simulink model "Copy_2_of_SUS_ST_GUI"  (R2013a)
settings: Solver=ode3  StartTime=0  StopTime=T  FixedStep=0.1  RelTol=1e-3
values from neighbouring files (symbols this model uses):
  CA = str2double(get(handles.CA,'string'))    [SUS_ST_0326.m]    (also in SUS_ST_GUI_0326.m)
  IN = str2double(get(handles.IN,'string'))    [SUS_ST_0326.m]    (also in SUS_ST_GUI_0326.m)
  LT = str2double(get(handles.LT,'string'))    [SUS_ST_GUI_0326.m]
  N = 1    [SUS_ST_0326.m]
  SR = str2double(get(handles.SR,'string'))    [SUS_ST_0326.m]    (also in SUS_ST_GUI_0326.m)
  ST = str2double(get(handles.ST,'string'))    [SUS_ST_GUI_0326.m]
  ST_S = str2double(get(handles.ST_S,'string'))    [SUS_ST_GUI_0326.m]
  T = 10    [SUS_ST_GUI_0326.m]
  T5 = str2double(get(handles.T5,'string'))    [SUS_ST_0326.m]    (also in SUS_ST_GUI_0326.m)
  T6 = str2double(get(handles.T6,'string'))    [SUS_ST_0326.m]    (also in SUS_ST_GUI_0326.m)
  X11 = (Z11-H/sind(CA)-b2_3)/k2_3    [SUS_ST_GUI_0326.m]
  X12 = (Z12-bb2_3)/k2_3    [SUS_ST_GUI_0326.m]
  X13 = X12-X12_3    [SUS_ST_GUI_0326.m]
  X14 = X9+X14_1    [SUS_ST_GUI_0326.m]
  X15 = X9+X15_1    [SUS_ST_GUI_0326.m]
  X16 = X9+X16_2    [SUS_ST_GUI_0326.m]
  X2 = -abs(Z3)*tand(CA)    [SUS_ST_GUI_0326.m]
  x2 = 0    [SUS_ST_GUI_0326.m]
  X3 = abs(Z2)*tand(CA)    [SUS_ST_GUI_0326.m]
  x3 = 0    [SUS_ST_GUI_0326.m]
  x4 = str2double(get(handles.x4,'string'))    [SUS_ST_0326.m]    (also in SUS_ST_GUI_0326.m)
  X5 = X4-a1*cosd(T5)    [SUS_ST_GUI_0326.m]
  x5 = 0    [SUS_ST_GUI_0326.m]
  X6 = X4+b1*cosd(T5)    [SUS_ST_GUI_0326.m]
  x6 = str2double(get(handles.x6,'string'))    [SUS_ST_0326.m]    (also in SUS_ST_GUI_0326.m)
  X7 = X1-a2*cosd(T6)    [SUS_ST_GUI_0326.m]
  x7 = x4-e7    [SUS_ST_GUI_0326.m]
  X8 = X1+b2*cosd(T6)    [SUS_ST_GUI_0326.m]
  x8 = x9-l8*sind(t8)    [SUS_ST_GUI_0326.m]
  X9 = str2double(get(handles.X9,'string'))    [SUS_ST_0326.m]    (also in SUS_ST_GUI_0326.m)
  x9 = str2double(get(handles.x9,'string'))    [SUS_ST_0326.m]    (also in SUS_ST_GUI_0326.m)
  XC1 = (X7+X2+X8)/3    [SUS_ST_GUI_0326.m]
  xc1 = (x3+x4+x5)/3    [SUS_ST_GUI_0326.m]
  XC2 = (X3+X2)/2    [SUS_ST_GUI_0326.m]
  XC3 = (X5+X3+X6)/3    [SUS_ST_GUI_0326.m]
  Y11 = M/2    [SUS_ST_GUI_0326.m]
  Y12 = (B11_12-BB2_3)/(K2_3-K11_12)    [SUS_ST_GUI_0326.m]
  Y13 = Y12-Y12_3    [SUS_ST_GUI_0326.m]
  Y14 = Y9+Y14_1    [SUS_ST_GUI_0326.m]
  Y15 = Y9+Y15_1    [SUS_ST_GUI_0326.m]
  Y16 = Y9+Y16_2    [SUS_ST_GUI_0326.m]
  Y2 = (Z2-Z9)/K2_3+Y9-SR    [SUS_ST_GUI_0326.m]
  y2 = Y1+l2*cosd(t2+T2)    [SUS_ST_GUI_0326.m]
  Y3 = (Z3-Z9)/K2_3+Y9-SR    [SUS_ST_GUI_0326.m]
  y3 = y4+l4*cosd(t4)    [SUS_ST_GUI_0326.m]
  y4 = str2double(get(handles.y4,'string'))    [SUS_ST_0326.m]    (also in SUS_ST_GUI_0326.m)
  Y5 = Y4    [SUS_ST_GUI_0326.m]
  y5 = y4+l5*cosd(t5)    [SUS_ST_GUI_0326.m]
  Y6 = Y4    [SUS_ST_GUI_0326.m]
  y6 = str2double(get(handles.y6,'string'))    [SUS_ST_0326.m]    (also in SUS_ST_GUI_0326.m)
  Y7 = Y1    [SUS_ST_GUI_0326.m]
  y7 = y4+l7*cosd(t7)    [SUS_ST_GUI_0326.m]
  Y8 = Y1    [SUS_ST_GUI_0326.m]
  y8 = y9+l8*cosd(t8)    [SUS_ST_GUI_0326.m]
  Y9 = str2double(get(handles.Y9,'string'))    [SUS_ST_0326.m]    (also in SUS_ST_GUI_0326.m)
  y9 = str2double(get(handles.y9,'string'))    [SUS_ST_0326.m]    (also in SUS_ST_GUI_0326.m)
  YC1 = (Y7+Y2+Y8)/3    [SUS_ST_GUI_0326.m]
  yc1 = (y3+y4+y5)/3    [SUS_ST_GUI_0326.m]
  YC2 = (Y3+Y2)/2    [SUS_ST_GUI_0326.m]
  YC3 = (Y5+Y3+Y6)/3    [SUS_ST_GUI_0326.m]
  Z11 = str2double(get(handles.Z11,'string'))    [SUS_ST_0326.m]    (also in SUS_ST_GUI_0326.m)
  Z12 = str2double(get(handles.Z12,'string'))    [SUS_ST_0326.m]    (also in SUS_ST_GUI_0326.m = K11_12*Y12+B11_12)
  Z13 = Z12-Z12_3    [SUS_ST_GUI_0326.m]
  Z14 = Z9+Z14_1    [SUS_ST_GUI_0326.m]
  Z15 = Z9+Z15_1    [SUS_ST_GUI_0326.m]
  Z16 = Z9+Z16_2    [SUS_ST_GUI_0326.m]
  Z2 = str2double(get(handles.Z2,'string'))    [SUS_ST_0326.m]    (also in SUS_ST_GUI_0326.m)
  z2 = Z1+l2*sind(t2+T2)    [SUS_ST_GUI_0326.m]
  Z3 = str2double(get(handles.Z3,'string'))    [SUS_ST_0326.m]    (also in SUS_ST_GUI_0326.m)
  z3 = z4+l4*sind(t4)    [SUS_ST_GUI_0326.m]
  z4 = str2double(get(handles.z4,'string'))    [SUS_ST_0326.m]    (also in SUS_ST_GUI_0326.m)
  Z5 = Z4-a1*sind(T5)    [SUS_ST_GUI_0326.m]
  z5 = z4+l5*sind(t5)    [SUS_ST_GUI_0326.m]
  Z6 = Z4+b1*sind(T5)    [SUS_ST_GUI_0326.m]
  z6 = str2double(get(handles.z6,'string'))    [SUS_ST_0326.m]    (also in SUS_ST_GUI_0326.m)
  Z7 = Z1-a2*sind(T6)    [SUS_ST_GUI_0326.m]
  z7 = z4+l7*sind(t7)    [SUS_ST_GUI_0326.m]
  Z8 = Z1+b2*sind(T6)    [SUS_ST_GUI_0326.m]
  z8 = z9    [SUS_ST_GUI_0326.m]
  Z9 = str2double(get(handles.Z9,'string'))    [SUS_ST_0326.m]    (also in SUS_ST_GUI_0326.m)
  z9 = str2double(get(handles.z9,'string'))    [SUS_ST_0326.m]    (also in SUS_ST_GUI_0326.m)
  ZC1 = (Z7+Z2+Z8)/3    [SUS_ST_GUI_0326.m]
  zc1 = (z3+z4+z5)/3    [SUS_ST_GUI_0326.m]
  ZC2 = (Z3+Z2)/2    [SUS_ST_GUI_0326.m]
  ZC3 = (Z5+Z3+Z6)/3    [SUS_ST_GUI_0326.m]
libraries: mblibv1 x77, simulink x3
(part 2 of 2)

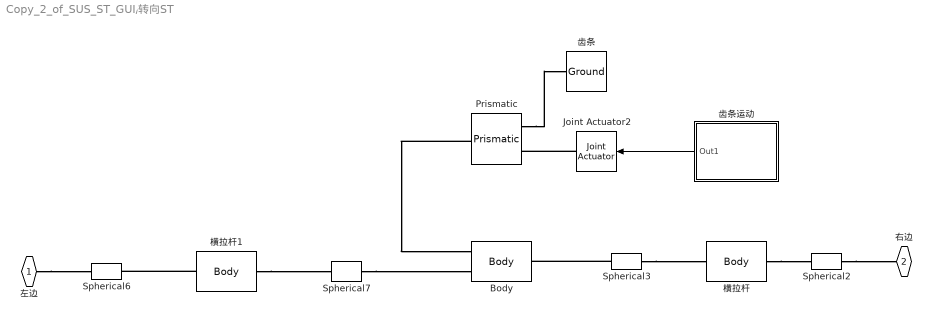
== system Copy_2_of_SUS_ST_GUI/转向ST ==
  Body : mblibv1/Bodies/Body  LConnTagsString=CG|CS1  RConnTagsString=CS2  UpdateFromCAD=off  DialogClass=MechanicalBodyBlock  Mass=1  MassUnits=kg  InertiaUnits=kg*m^2  Inertia=eye(3)  Shape=Cylinder  ShapeDims=[1 1]  ShapeUnits=m  ShapeUse=false  Density=1  DensityUnits=kg/m^3  DensityUse=false  GraphicsMode=MACHINE_DEFAULT  BodyColorSelMode=MACHINE_DEFAULT  BodyColor=[1 0 0]  AttachedToCS=CG  CG=Left$CG$[X11 0 Z11]$WORLD$WORLD$mm$[0 0 0]$Euler X-Y-Z$deg$WORLD$true$none  WorkingFrames=Left$CS1$[X11 -Y11 Z11]$World$World$mm$[0 0 0]$Euler X-Y-Z$deg$WORLD$true$none#Right$CS2$[X11 Y11 Z11]$World$World$mm$[0 0 0]$Euler X-Y-Z$deg$WORLD$true$none  CGPos=[X11 0 Z11]  CGRot=[0 0 0]  CS0Pos=[]  CS0Rot=[]  CS1Pos=[X11 -Y11 Z11]  CS1Rot=[0 0 0]  CS2Pos=[X11 Y11 Z11]  CS2Rot=[0 0 0]  CS3Pos=[]  CS3Rot=[]  CS4Pos=[]  CS4Rot=[]  CS5Pos=[]  CS5Rot=[]  CS6Pos=[]  CS6Rot=[]  CS7Pos=[]  CS7Rot=[]  CS8Pos=[]  CS8Rot=[]  CS9Pos=[]  CS9Rot=[]  CS10Pos=[]  CS10Rot=[]  CS11Pos=[]  CS11Rot=[]  CS12Pos=[]  CS12Rot=[]  CS13Pos=[]  CS13Rot=[]  CS14Pos=[]  CS14Rot=[]  CS15Pos=[]  CS15Rot=[]  CS16Pos=[]  CS16Rot=[]  CS17Pos=[]  CS17Rot=[]  CS18Pos=[]  CS18Rot=[]  CS19Pos=[]  CS19Rot=[]  CS20Pos=[]  CS20Rot=[]
  Joint Actuator2 : mblibv1/Sensors &  Actuators/Joint Actuator  UpdateFromCAD=off  PhysicalDomain=Mechanical  PortType=blob  ActuationStyle=Motion  AngleUnits=deg  ArcVelocityUnits=deg/s  ArcAccelerationUnits=deg/s^2  CoordPositionUnits=mm  VelocityUnits=mm/s  AccelerationUnits=mm/s^2  ForceUnits=N  TorqueUnits=N*m  ActiveIO=on  Width=3  DialogClass=MechanicalActuatorBlock  Primitive=P1  ReferenceFrame=Absolute (World)
  Prismatic : mblibv1/Joints/Prismatic  LConnTagsString=__newl0|SA1  RConnTagsString=__newr0  UpdateFromCAD=off  NumSAPorts=1  CutJoint=off  MarkAsCut=off  Primitives=prismatic  PrimitiveProps=P1$World$[0 1 0]$prismatic  DialogClass=JointBlock  P1Axis=[0 1 0]
  Spherical{2..3,6..7} (4 alike) : mblibv1/Joints/Spherical  LConnTagsString=__newl0  RConnTagsString=__newr0  UpdateFromCAD=off  NumSAPorts=0  CutJoint=off  MarkAsCut=off  Primitives=spherical  PrimitiveProps=S$WORLD$[0 0 0]$spherical  DialogClass=JointBlock  SAxis=[0 0 0]
  横拉杆 : mblibv1/Bodies/Body  LConnTagsString=CS1  RConnTagsString=CS2  UpdateFromCAD=off  DialogClass=MechanicalBodyBlock  Mass=1  MassUnits=kg  InertiaUnits=kg*m^2  Inertia=eye(3)  Shape=Cylinder  ShapeDims=[1 1]  ShapeUnits=m  ShapeUse=false  Density=1  DensityUnits=kg/m^3  DensityUse=false  GraphicsMode=MACHINE_DEFAULT  BodyColorSelMode=MACHINE_DEFAULT  BodyColor=[1 0 0]  AttachedToCS=CG  CG=Left$CG$[(X11+X12)/2 (Y11+Y12)/2 (Z11+Z12)/2]$WORLD$WORLD$mm$[0 0 0]$Euler X-Y-Z$deg$WORLD$false$none  WorkingFrames=Left$CS1$[X11 Y11 Z11]$World$World$mm$[0 0 0]$Euler X-Y-Z$deg$WORLD$true$none#Right$CS2$[X12 Y12 Z12]$World$World$mm$[0 0 0]$Euler X-Y-Z$deg$WORLD$true$none  CGPos=[(X11+X12)/2 (Y11+Y12)/2 (Z11+Z12)/2]  CGRot=[0 0 0]  CS0Pos=[]  CS0Rot=[]  CS1Pos=[X11 Y11 Z11]  CS1Rot=[0 0 0]  CS2Pos=[X12 Y12 Z12]  CS2Rot=[0 0 0]  CS3Pos=[]  CS3Rot=[]  CS4Pos=[]  CS4Rot=[]  CS5Pos=[]  CS5Rot=[]  CS6Pos=[]  CS6Rot=[]  CS7Pos=[]  CS7Rot=[]  CS8Pos=[]  CS8Rot=[]  CS9Pos=[]  CS9Rot=[]  CS10Pos=[]  CS10Rot=[]  CS11Pos=[]  CS11Rot=[]  CS12Pos=[]  CS12Rot=[]  CS13Pos=[]  CS13Rot=[]  CS14Pos=[]  CS14Rot=[]  CS15Pos=[]  CS15Rot=[]  CS16Pos=[]  CS16Rot=[]  CS17Pos=[]  CS17Rot=[]  CS18Pos=[]  CS18Rot=[]  CS19Pos=[]  CS19Rot=[]  CS20Pos=[]  CS20Rot=[]
  横拉杆1 : mblibv1/Bodies/Body  LConnTagsString=CS1  RConnTagsString=CS2  UpdateFromCAD=off  DialogClass=MechanicalBodyBlock  Mass=1  MassUnits=kg  InertiaUnits=kg*m^2  Inertia=eye(3)  Shape=Cylinder  ShapeDims=[1 1]  ShapeUnits=m  ShapeUse=false  Density=1  DensityUnits=kg/m^3  DensityUse=false  GraphicsMode=MACHINE_DEFAULT  BodyColorSelMode=MACHINE_DEFAULT  BodyColor=[1 0 0]  AttachedToCS=CG  CG=Left$CG$[(X11+X12)/2 -(Y11+Y12)/2 (Z11+Z12)/2]$WORLD$WORLD$mm$[0 0 0]$Euler X-Y-Z$deg$WORLD$false$none  WorkingFrames=Left$CS1$[X11 -Y11 Z11]$World$World$mm$[0 0 0]$Euler X-Y-Z$deg$WORLD$true$none#Right$CS2$[X12 -Y12 Z12]$World$World$mm$[0 0 0]$Euler X-Y-Z$deg$WORLD$true$none  CGPos=[(X11+X12)/2 -(Y11+Y12)/2 (Z11+Z12)/2]  CGRot=[0 0 0]  CS0Pos=[]  CS0Rot=[]  CS1Pos=[X11 -Y11 Z11]  CS1Rot=[0 0 0]  CS2Pos=[X12 -Y12 Z12]  CS2Rot=[0 0 0]  CS3Pos=[]  CS3Rot=[]  CS4Pos=[]  CS4Rot=[]  CS5Pos=[]  CS5Rot=[]  CS6Pos=[]  CS6Rot=[]  CS7Pos=[]  CS7Rot=[]  CS8Pos=[]  CS8Rot=[]  CS9Pos=[]  CS9Rot=[]  CS10Pos=[]  CS10Rot=[]  CS11Pos=[]  CS11Rot=[]  CS12Pos=[]  CS12Rot=[]  CS13Pos=[]  CS13Rot=[]  CS14Pos=[]  CS14Rot=[]  CS15Pos=[]  CS15Rot=[]  CS16Pos=[]  CS16Rot=[]  CS17Pos=[]  CS17Rot=[]  CS18Pos=[]  CS18Rot=[]  CS19Pos=[]  CS19Rot=[]  CS20Pos=[]  CS20Rot=[]
  齿条 : mblibv1/Bodies/Ground  UpdateFromCAD=off  LeftPortType=env  RightPortType=workingframe  PhysicalDomain=Mechanical  DialogClass=GroundBlock  CoordPosition=[X11 0 Z11]  CoordPositionUnits=mm  StateVectorMgrId=-1  MachineId=[0 0]  ShowEnvPort=off
  齿条运动 : Subsystem
  左边 : PMIOPort  Port=1  Side=Left
  右边 : PMIOPort  Port=2  Side=Right
  wires:
  齿条运动/1(Out1) -> Joint Actuator2/1
  connections:
  Spherical7/RConn1 -- Body/LConn2
  横拉杆/RConn1 -- Spherical2/LConn1
  左边/RConn1 -- Spherical6/RConn1
  Spherical2/RConn1 -- 右边/RConn1
  Spherical3/LConn1 -- Body/RConn1
  横拉杆1/LConn1 -- Spherical7/LConn1
  Prismatic/RConn1 -- Body/LConn1
  Prismatic/LConn1 -- 齿条/RConn1
  Joint Actuator2/RConn1 -- Prismatic/LConn2
  Spherical3/RConn1 -- 横拉杆/LConn1
  横拉杆1/RConn1 -- Spherical6/LConn1

== system Copy_2_of_SUS_ST_GUI/右摇臂推杆/5 ==
  In1 : Inport
  Demux : Demux  Outputs=3
  To Workspace : ToWorkspace  VariableName=x5  SampleTime=-1
  To Workspace1 : ToWorkspace  VariableName=y5  SampleTime=-1
  To Workspace2 : ToWorkspace  VariableName=z5  SampleTime=-1
  wires:
  Demux/2 -> To Workspace1/1
  Demux/1 -> To Workspace/1
  Demux/3 -> To Workspace2/1
  In1/1 -> Demux/1

== system Copy_2_of_SUS_ST_GUI/右测量/12坐标 ==
  In1 : Inport
  Demux : Demux  Outputs=3
  To Workspace : ToWorkspace  VariableName=X12  SampleTime=-1
  To Workspace1 : ToWorkspace  VariableName=Y12  SampleTime=-1
  To Workspace2 : ToWorkspace  VariableName=Z12  SampleTime=-1
  wires:
  Demux/2 -> To Workspace1/1
  Demux/1 -> To Workspace/1
  Demux/3 -> To Workspace2/1
  In1/1 -> Demux/1

== system Copy_2_of_SUS_ST_GUI/右测量/13坐标 ==
  In1 : Inport
  Demux : Demux  Outputs=3
  To Workspace : ToWorkspace  VariableName=X13  SampleTime=-1
  To Workspace1 : ToWorkspace  VariableName=Y13  SampleTime=-1
  To Workspace2 : ToWorkspace  VariableName=Z13  SampleTime=-1
  wires:
  Demux/2 -> To Workspace1/1
  Demux/1 -> To Workspace/1
  Demux/3 -> To Workspace2/1
  In1/1 -> Demux/1

== system Copy_2_of_SUS_ST_GUI/右测量/14坐标1 ==
  In1 : Inport
  Demux : Demux  Outputs=3
  To Workspace : ToWorkspace  VariableName=X14  SampleTime=-1
  To Workspace1 : ToWorkspace  VariableName=Y14  SampleTime=-1
  To Workspace2 : ToWorkspace  VariableName=Z14  SampleTime=-1
  wires:
  In1/1 -> Demux/1
  Demux/3 -> To Workspace2/1
  Demux/1 -> To Workspace/1
  Demux/2 -> To Workspace1/1

== system Copy_2_of_SUS_ST_GUI/右测量/15坐标2 ==
  In1 : Inport
  Demux : Demux  Outputs=3
  To Workspace : ToWorkspace  VariableName=X15  SampleTime=-1
  To Workspace1 : ToWorkspace  VariableName=Y15  SampleTime=-1
  To Workspace2 : ToWorkspace  VariableName=Z15  SampleTime=-1
  wires:
  Demux/2 -> To Workspace1/1
  Demux/1 -> To Workspace/1
  Demux/3 -> To Workspace2/1
  In1/1 -> Demux/1

== system Copy_2_of_SUS_ST_GUI/右测量/16坐标1 ==
  In1 : Inport
  Demux : Demux  Outputs=3
  To Workspace : ToWorkspace  VariableName=X16  SampleTime=-1
  To Workspace1 : ToWorkspace  VariableName=Y16  SampleTime=-1
  To Workspace2 : ToWorkspace  VariableName=Z16  SampleTime=-1
  wires:
  In1/1 -> Demux/1
  Demux/3 -> To Workspace2/1
  Demux/1 -> To Workspace/1
  Demux/2 -> To Workspace1/1

== system Copy_2_of_SUS_ST_GUI/右测量/2坐标 ==
  In1 : Inport
  Demux : Demux  Outputs=3
  To Workspace : ToWorkspace  VariableName=X2  SampleTime=-1
  To Workspace1 : ToWorkspace  VariableName=Y2  SampleTime=-1
  To Workspace2 : ToWorkspace  VariableName=Z2  SampleTime=-1
  wires:
  Demux/2 -> To Workspace1/1
  Demux/1 -> To Workspace/1
  Demux/3 -> To Workspace2/1
  In1/1 -> Demux/1

== system Copy_2_of_SUS_ST_GUI/右测量/3坐标 ==
  In1 : Inport
  Demux : Demux  Outputs=3
  To Workspace : ToWorkspace  VariableName=X3  SampleTime=-1
  To Workspace1 : ToWorkspace  VariableName=Y3  SampleTime=-1
  To Workspace2 : ToWorkspace  VariableName=Z3  SampleTime=-1
  wires:
  In1/1 -> Demux/1
  Demux/3 -> To Workspace2/1
  Demux/1 -> To Workspace/1
  Demux/2 -> To Workspace1/1

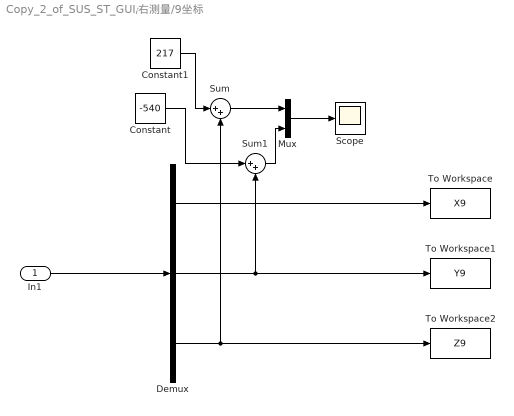
== system Copy_2_of_SUS_ST_GUI/右测量/9坐标 ==
  In1 : Inport
  Constant : Constant  Value=-540
  Constant1 : Constant  Value=217
  Demux : Demux  Outputs=3
  Mux : Mux  Inputs=2
  Scope : Scope
      settings: TimeRange=10  YMin=-0.5  YMax=1
  Sum : Sum  Inputs=|++
  Sum1 : Sum  Inputs=|++
  To Workspace : ToWorkspace  VariableName=X9  SampleTime=-1
  To Workspace1 : ToWorkspace  VariableName=Y9  SampleTime=-1
  To Workspace2 : ToWorkspace  VariableName=Z9  SampleTime=-1
  wires:
  Demux/2 -> To Workspace1/1, Sum1/2
  Demux/1 -> To Workspace/1
  Demux/3 -> Sum/2, To Workspace2/1
  In1/1 -> Demux/1
  Mux/1 -> Scope/1
  Sum/1 -> Mux/1
  Sum1/1 -> Mux/2
  Constant1/1 -> Sum/1
  Constant/1 -> Sum1/1

== system Copy_2_of_SUS_ST_GUI/左测量/12' ==
  In1 : Inport
  Demux : Demux  Outputs=3
  To Workspace : ToWorkspace  VariableName=X_12  SampleTime=-1
  To Workspace1 : ToWorkspace  VariableName=Y_12  SampleTime=-1
  To Workspace2 : ToWorkspace  VariableName=Z_12  SampleTime=-1
  wires:
  In1/1 -> Demux/1
  Demux/3 -> To Workspace2/1
  Demux/1 -> To Workspace/1
  Demux/2 -> To Workspace1/1

== system Copy_2_of_SUS_ST_GUI/左测量/13坐标 ==
  In1 : Inport
  Demux : Demux  Outputs=3
  To Workspace : ToWorkspace  VariableName=X_13  SampleTime=-1
  To Workspace1 : ToWorkspace  VariableName=Y_13  SampleTime=-1
  To Workspace2 : ToWorkspace  VariableName=Z_13  SampleTime=-1
  wires:
  In1/1 -> Demux/1
  Demux/3 -> To Workspace2/1
  Demux/1 -> To Workspace/1
  Demux/2 -> To Workspace1/1

== system Copy_2_of_SUS_ST_GUI/左测量/14坐标1 ==
  In1 : Inport
  Demux : Demux  Outputs=3
  To Workspace : ToWorkspace  VariableName=X_14  SampleTime=-1
  To Workspace1 : ToWorkspace  VariableName=Y_14  SampleTime=-1
  To Workspace2 : ToWorkspace  VariableName=Z_14  SampleTime=-1
  wires:
  In1/1 -> Demux/1
  Demux/3 -> To Workspace2/1
  Demux/1 -> To Workspace/1
  Demux/2 -> To Workspace1/1

== system Copy_2_of_SUS_ST_GUI/左测量/15坐标2 ==
  In1 : Inport
  Demux : Demux  Outputs=3
  To Workspace : ToWorkspace  VariableName=X_15  SampleTime=-1
  To Workspace1 : ToWorkspace  VariableName=Y_15  SampleTime=-1
  To Workspace2 : ToWorkspace  VariableName=Z_15  SampleTime=-1
  wires:
  Demux/2 -> To Workspace1/1
  Demux/1 -> To Workspace/1
  Demux/3 -> To Workspace2/1
  In1/1 -> Demux/1

== system Copy_2_of_SUS_ST_GUI/左测量/16坐标1 ==
  In1 : Inport
  Demux : Demux  Outputs=3
  To Workspace : ToWorkspace  VariableName=X_16  SampleTime=-1
  To Workspace1 : ToWorkspace  VariableName=Y_16  SampleTime=-1
  To Workspace2 : ToWorkspace  VariableName=Z_16  SampleTime=-1
  wires:
  In1/1 -> Demux/1
  Demux/3 -> To Workspace2/1
  Demux/1 -> To Workspace/1
  Demux/2 -> To Workspace1/1

== system Copy_2_of_SUS_ST_GUI/左测量/9 ==
  In1 : Inport
  Demux : Demux  Outputs=3
  Scope : Scope
      settings: TimeRange=10  YMin=-0.5  YMax=1
  To Workspace : ToWorkspace  VariableName=X_9  SampleTime=-1
  To Workspace1 : ToWorkspace  VariableName=Y_9  SampleTime=-1
  To Workspace2 : ToWorkspace  VariableName=Z_9  SampleTime=-1
  wires:
  In1/1 -> Demux/1
  Demux/3 -> To Workspace2/1
  Demux/1 -> To Workspace/1
  Demux/2 -> To Workspace1/1, Scope/1

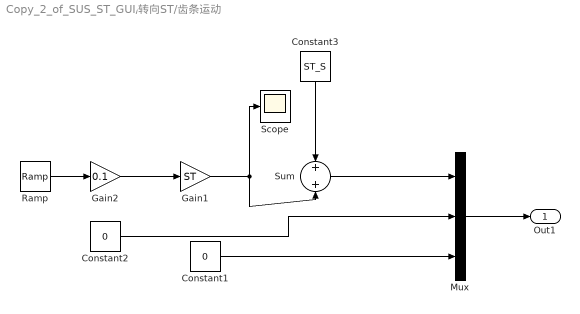
== system Copy_2_of_SUS_ST_GUI/转向ST/齿条运动 ==
  Constant1 : Constant  Value=0
  Constant2 : Constant  Value=0
  Constant3 : Constant  Value=ST_S
  Gain1 : Gain  Gain=ST
  Gain2 : Gain  Gain=0.1
  Mux : Mux  Inputs=3
  Ramp : simulink/Sources/Ramp  slope=1  start=0  X0=0
  Scope : Scope
      settings: TimeRange=10  YMin=-0.5  YMax=1
  Sum : Sum  Inputs=+|+
  Out1 : Outport
  wires:
  Ramp/1 -> Gain2/1
  Constant2/1 -> Mux/2
  Constant1/1 -> Mux/3
  Mux/1 -> Out1/1
  Gain1/1 -> Sum/2, Scope/1
  Gain2/1 -> Gain1/1
  Sum/1 -> Mux/1
  Constant3/1 -> Sum/1
